simulink model "TIM"  (R2017b)
settings: Solver=ode45  StartTime=0.0  StopTime=inf  RelTol=1e-3
undefined symbols (not defined in the file): sigbuilder_block
(part 1 of 2)
settings Model: Creator=matlab01  LastModifiedBy=matlab01

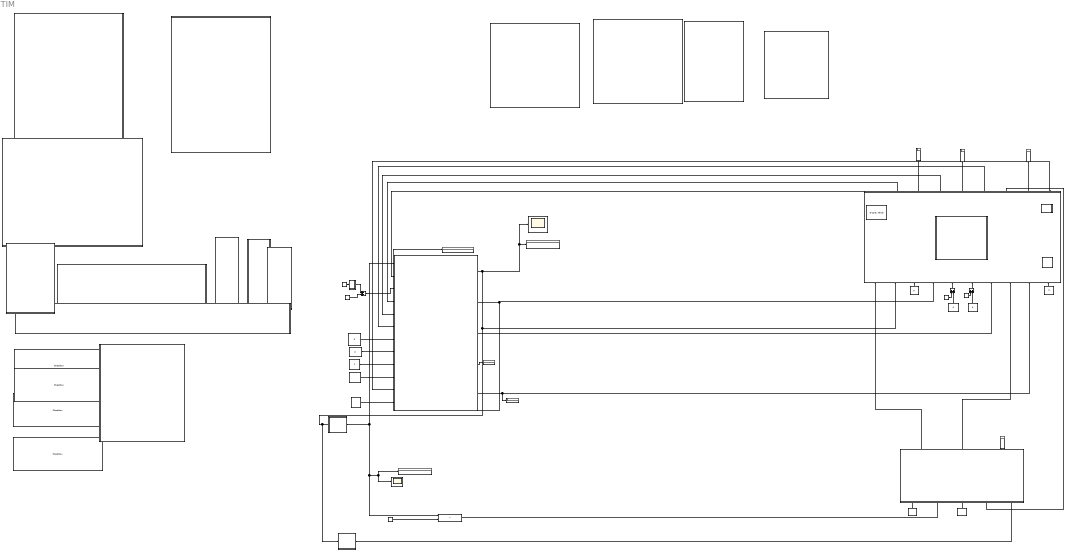
== system TIM ==
  note: Subsystem
  note: Subsystem
  Add : Sum
  Add1 : Sum
  Add2 : Sum
  Bale Pass Sr : Constant  Value=0
  Bale Size Sr : Constant  Value=0
  Baler : Subsystem
  Baler Stopped : Subsystem  DialogController=hmiCreateDDGDialog  IsWebBlock=on  mask(MWDashboardBlock){webBlockId=380f0481-0464-4552-ac21-b39f29efcae4, webBlockType=lamp, ShowInLibBrowser=on, ShowInitialText=on, HMISrcModelName=TIM}
      mask prompts: webBlockType "WebBlock Type"; HMISrcModelName "Source Model"
      mask help: SimulinkHMI:dialogs:LampDialogDesc
      mask Help: helpview([docroot '/mapfiles/simulink.map'], 'hmi_lamp')
      mask Display:
      | if strcmp(get_param(bdroot(gcb),'BlockDiagramType'), 'library')
      |     image([(matlabroot) '/toolbox/simulink/hmi/icons/Lamp.png']);
      | end
  BalerCFG : DisplayBlock  WebBlockId=422  ModelName=TIM  LabelPosition=Hide  ShowInitialText=on  ShowFormattedStrings=off  Format=long  Alignment=Center
  CFG : Display
  Check Box : Checkbox  WebBlockId=680  ModelName=TIM  LabelPosition=Hide  ShowInitialText=off  Checked=on  Label=RearSr_1_Fail
  Check Box1 : Checkbox  WebBlockId=681  ModelName=TIM  LabelPosition=Hide  ShowInitialText=off  Checked=on  Label=RearSr_2_Fail
  Check Box2 : Checkbox  WebBlockId=682  ModelName=TIM  LabelPosition=Hide  ShowInitialText=off  Checked=off  Label=SpeedSr_Fail
  Check Box3 : Checkbox  WebBlockId=683  ModelName=TIM  LabelPosition=Hide  ShowInitialText=off  Checked=off  Label=FrontObstSr_Fail
  Constant : Constant  Value=2
  Constant1 : Constant  Value=2
  Display{,1..2,4..6} (6 alike) : Display
  Display3 : DisplayBlock  WebBlockId=427  ModelName=TIM  LabelPosition=Hide  ShowInitialText=on  ShowFormattedStrings=off  Format=long  Alignment=Center
  Display7 : DisplayBlock  WebBlockId=429  ModelName=TIM  LabelPosition=Hide  ShowInitialText=on  ShowFormattedStrings=off  Format=long  Alignment=Center
  DoorStatus : Display
  Front Obstacle : Constant  Value=0
  FrontObstSr : Subsystem
  FrontObstSrFail : Constant  Value=0
  Gauge : Subsystem  DialogController=hmiCreateDDGDialog  IsWebBlock=on  mask(MWDashboardBlock){webBlockId=a8481909-2d34-4551-932e-729d5791eb58, webBlockType=circulargauge, ShowInLibBrowser=on, ShowInitialText=on, HMISrcModelName=TIM}
      mask prompts: webBlockId "WebBlock Id"; webBlockType "WebBlock Type"; HMISrcModelName "Source Model"
      mask help: SimulinkHMI:dialogs:CircularGaugeDialogDesc
      mask Help: helpview([docroot '/mapfiles/simulink.map'], 'hmi_gauge')
      mask Display:
      | if strcmp(get_param(bdroot(gcb),'BlockDiagramType'), 'library')
      |     image([(matlabroot) '/toolbox/simulink/hmi/icons/CircularGauge.png']);
      | end
  Half Gauge : Subsystem  DialogController=hmiCreateDDGDialog  IsWebBlock=on  mask(MWDashboardBlock){webBlockId=1767aec4-c0de-4876-b9ef-c44c12ba7e5c, webBlockType=semicirculargauge, ShowInLibBrowser=on, ShowInitialText=on, HMISrcModelName=TIM}
      mask prompts: webBlockId "WebBlock Id"; webBlockType "WebBlock Type"; HMISrcModelName "Source Model"
      mask help: SimulinkHMI:dialogs:SemicircularGaugeDialogDesc
      mask Help: helpview([docroot '/mapfiles/simulink.map'], 'hmi_half_gauge')
      mask Display:
      | if strcmp(get_param(bdroot(gcb),'BlockDiagramType'), 'library')
      |     image([(matlabroot) '/toolbox/simulink/hmi/icons/SemicircularGauge.png']);
      | end
  Knob : Subsystem  DialogController=hmiCreateDDGDialog  IsWebBlock=on  mask(MWDashboardBlock){webBlockId=44b2cfbf-7851-438f-9afd-65227a1c2716, webBlockType=continuousknob, ShowInLibBrowser=on, ShowInitialText=on, HMISrcModelName=TIM}
      mask prompts: webBlockId "WebBlock Id"; webBlockType "WebBlock Type"; HMISrcModelName "Source Model"
      mask help: SimulinkHMI:dialogs:ContinuousKnobDialogDesc
      mask Help: helpview([docroot '/mapfiles/simulink.map'], 'hmi_knob')
      mask Display:
      | if strcmp(get_param(bdroot(gcb),'BlockDiagramType'), 'library')
      |     image([(matlabroot) '/toolbox/simulink/hmi/icons/ContinuousKnob.png']);
      | end
  Knob1 : Subsystem  DialogController=hmiCreateDDGDialog  IsWebBlock=on  mask(MWDashboardBlock){webBlockId=555d5953-f540-48b0-b281-3241b1506ee0, webBlockType=continuousknob, ShowInLibBrowser=on, ShowInitialText=on, HMISrcModelName=TIM}
      mask prompts: webBlockId "WebBlock Id"; webBlockType "WebBlock Type"; HMISrcModelName "Source Model"
      mask help: SimulinkHMI:dialogs:ContinuousKnobDialogDesc
      mask Help: helpview([docroot '/mapfiles/simulink.map'], 'hmi_knob')
      mask Display:
      | if strcmp(get_param(bdroot(gcb),'BlockDiagramType'), 'library')
      |     image([(matlabroot) '/toolbox/simulink/hmi/icons/ContinuousKnob.png']);
      | end
  Lamp : Subsystem  DialogController=hmiCreateDDGDialog  IsWebBlock=on  mask(MWDashboardBlock){webBlockId=33d9c165-8687-4e0a-bfea-f4d86ec876ec, webBlockType=lamp, ShowInLibBrowser=on, ShowInitialText=on, HMISrcModelName=TIM}
      mask prompts: webBlockType "WebBlock Type"; HMISrcModelName "Source Model"
      mask help: SimulinkHMI:dialogs:LampDialogDesc
      mask Help: helpview([docroot '/mapfiles/simulink.map'], 'hmi_lamp')
      mask Display:
      | if strcmp(get_param(bdroot(gcb),'BlockDiagramType'), 'library')
      |     image([(matlabroot) '/toolbox/simulink/hmi/icons/Lamp.png']);
      | end
  Lamp1 : Subsystem  DialogController=hmiCreateDDGDialog  IsWebBlock=on  mask(MWDashboardBlock){webBlockId=c492ce9b-3337-4b76-9797-8f79f533d9ec, webBlockType=lamp, ShowInLibBrowser=on, ShowInitialText=on, HMISrcModelName=TIM}
      mask prompts: webBlockType "WebBlock Type"; HMISrcModelName "Source Model"
      mask help: SimulinkHMI:dialogs:LampDialogDesc
      mask Help: helpview([docroot '/mapfiles/simulink.map'], 'hmi_lamp')
      mask Display:
      | if strcmp(get_param(bdroot(gcb),'BlockDiagramType'), 'library')
      |     image([(matlabroot) '/toolbox/simulink/hmi/icons/Lamp.png']);
      | end
  Product : Product
  RearDoor : Subsystem  DialogController=hmiCreateDDGDialog  IsWebBlock=on  mask(MWDashboardBlock){webBlockId=b538fc73-89be-495c-b7c3-b8c3e3397391, webBlockType=lamp, ShowInLibBrowser=on, ShowInitialText=on, HMISrcModelName=TIM}
      mask prompts: webBlockType "WebBlock Type"; HMISrcModelName "Source Model"
      mask help: SimulinkHMI:dialogs:LampDialogDesc
      mask Help: helpview([docroot '/mapfiles/simulink.map'], 'hmi_lamp')
      mask Display:
      | if strcmp(get_param(bdroot(gcb),'BlockDiagramType'), 'library')
      |     image([(matlabroot) '/toolbox/simulink/hmi/icons/Lamp.png']);
      | end
  RearObstSr : Subsystem  DialogController=hmiCreateDDGDialog  IsWebBlock=on  mask(MWDashboardBlock){webBlockId=2f04e0dc-cfdf-4b89-b502-650f31ce5fe2, webBlockType=rockerswitch, ShowInLibBrowser=on, ShowInitialText=on, HMISrcModelName=TIM}
      mask prompts: webBlockId "WebBlock Id"; webBlockType "WebBlock Type"; HMISrcModelName "Source Model"
      mask help: SimulinkHMI:dialogs:SwitchDialogDesc
      mask Help: helpview([docroot '/mapfiles/simulink.map'], 'hmi_rocker_switch')
      mask Display:
      | if strcmp(get_param(bdroot(gcb),'BlockDiagramType'), 'library')
      |     image([(matlabroot) '/toolbox/simulink/hmi/icons/RockerSwitch.png']);
      | end
  RearObstSr1 : Subsystem  DialogController=hmiCreateDDGDialog  IsWebBlock=on  mask(MWDashboardBlock){webBlockId=c64d6447-8e55-46e9-b568-5078a23053e9, webBlockType=rockerswitch, ShowInLibBrowser=on, ShowInitialText=on, HMISrcModelName=TIM}
      mask prompts: webBlockId "WebBlock Id"; webBlockType "WebBlock Type"; HMISrcModelName "Source Model"
      mask help: SimulinkHMI:dialogs:SwitchDialogDesc
      mask Help: helpview([docroot '/mapfiles/simulink.map'], 'hmi_rocker_switch')
      mask Display:
      | if strcmp(get_param(bdroot(gcb),'BlockDiagramType'), 'library')
      |     image([(matlabroot) '/toolbox/simulink/hmi/icons/RockerSwitch.png']);
      | end
  RearObstSr2 : Subsystem  DialogController=hmiCreateDDGDialog  IsWebBlock=on  mask(MWDashboardBlock){webBlockId=c4afeddd-f4a6-4f0c-9e01-adb611532535, webBlockType=rockerswitch, ShowInLibBrowser=on, ShowInitialText=on, HMISrcModelName=TIM}
      mask prompts: webBlockId "WebBlock Id"; webBlockType "WebBlock Type"; HMISrcModelName "Source Model"
      mask help: SimulinkHMI:dialogs:SwitchDialogDesc
      mask Help: helpview([docroot '/mapfiles/simulink.map'], 'hmi_rocker_switch')
      mask Display:
      | if strcmp(get_param(bdroot(gcb),'BlockDiagramType'), 'library')
      |     image([(matlabroot) '/toolbox/simulink/hmi/icons/RockerSwitch.png']);
      | end
  RearSr1 : Constant  Value=0
  RearSr2 : Constant  Value=0
  Rotary Switch : Subsystem  DialogController=hmiCreateDDGDialog  IsWebBlock=on  mask(MWDashboardBlock){webBlockId=4718e849-02b3-481c-8935-c4c34f11cecd, webBlockType=discreteknob, ShowInLibBrowser=on, ShowInitialText=on, HMISrcModelName=TIM}
      mask prompts: webBlockId "WebBlock Id"; webBlockType "WebBlock Type"; HMISrcModelName "Source Model"
      mask help: SimulinkHMI:dialogs:DiscreteKnobDialogDesc
      mask Help: helpview([docroot '/mapfiles/simulink.map'], 'hmi_rotary_switch')
      mask Display:
      | model = bdroot(gcb);
      | if strcmp(get_param(model,'BlockDiagramType'), 'library')
      |     image([(matlabroot) '/toolbox/simulink/hmi/icons/DiscreteKnob.png']);
      | end
  Rotary Switch1 : Subsystem  DialogController=hmiCreateDDGDialog  IsWebBlock=on  mask(MWDashboardBlock){webBlockId=f404cd82-44b9-4011-b588-6289506ab41c, webBlockType=discreteknob, ShowInLibBrowser=on, ShowInitialText=on, HMISrcModelName=TIM}
      mask prompts: webBlockId "WebBlock Id"; webBlockType "WebBlock Type"; HMISrcModelName "Source Model"
      mask help: SimulinkHMI:dialogs:DiscreteKnobDialogDesc
      mask Help: helpview([docroot '/mapfiles/simulink.map'], 'hmi_rotary_switch')
      mask Display:
      | model = bdroot(gcb);
      | if strcmp(get_param(model,'BlockDiagramType'), 'library')
      |     image([(matlabroot) '/toolbox/simulink/hmi/icons/DiscreteKnob.png']);
      | end
  Rotary Switch3 : Subsystem  DialogController=hmiCreateDDGDialog  IsWebBlock=on  mask(MWDashboardBlock){webBlockId=10fa69e3-8ad0-4a7e-b427-115ef8b6ee24, webBlockType=discreteknob, ShowInLibBrowser=on, ShowInitialText=on, HMISrcModelName=TIM}
      mask prompts: webBlockId "WebBlock Id"; webBlockType "WebBlock Type"; HMISrcModelName "Source Model"
      mask help: SimulinkHMI:dialogs:DiscreteKnobDialogDesc
      mask Help: helpview([docroot '/mapfiles/simulink.map'], 'hmi_rotary_switch')
      mask Display:
      | model = bdroot(gcb);
      | if strcmp(get_param(model,'BlockDiagramType'), 'library')
      |     image([(matlabroot) '/toolbox/simulink/hmi/icons/DiscreteKnob.png']);
      | end
  Scope : Scope
  Scope1 : Scope
  SettedSpeed : Display
  Slider : Subsystem  DialogController=hmiCreateDDGDialog  IsWebBlock=on  mask(MWDashboardBlock){webBlockId=15a6815c-0950-4bd8-89d9-de0febee8296, webBlockType=slider, ShowInLibBrowser=on, ShowInitialText=on, HMISrcModelName=TIM}
      mask prompts: webBlockId "WebBlock Id"; webBlockType "WebBlock Type"; HMISrcModelName "Source Model"
      mask help: SimulinkHMI:dialogs:SliderDialogDesc
      mask Help: helpview([docroot '/mapfiles/simulink.map'], 'hmi_slider')
      mask Display:
      | if strcmp(get_param(bdroot(gcb),'BlockDiagramType'), 'library')
      |     image([(matlabroot) '/toolbox/simulink/hmi/icons/Slider.png']);
      | end
  SpSr1Fail : Constant
  "SpeedSr1 " : Subsystem
  SpeedSr2,3 : Subsystem
  SpeedUserInput : Constant  Value=1.6036611567786
  SteeringUserInput : Constant  Value=-8.201570129395
  StopUserCMD : Constant  Value=0
  Swath  Area : Subsystem  DialogController=hmiCreateDDGDialog  IsWebBlock=on  mask(MathWorksWebBlock){webBlockId=664e3edd-25bd-4079-b9dd-da0d72c7846e, webBlockType=continuousknob, ShowInLibBrowser=on, ShowInitialText=on, HMISrcModelName=TIM}
      mask prompts: webBlockId "WebBlock Id"; webBlockType "WebBlock Type"; HMISrcModelName "Source Model"
      mask Help: helpview([docroot '/mapfiles/simulink.map'], 'hmi_knob')
      mask Display:
      | if strcmp(get_param(bdroot(gcb),'BlockDiagramType'), 'library')
      |     image([(matlabroot) '/toolbox/simulink/hmi/icons/ContinuousKnob.png']);
      | end
  Swath Area Value : Constant  Value=4.4148442586263
  SwathLocationSr : Constant  Value=-1.61220043573
  SwathScanner : Subsystem
  SysMode : Constant  Value=3
  Toggle Switch : Subsystem  DialogController=hmiCreateDDGDialog  IsWebBlock=on  mask(MWDashboardBlock){webBlockId=ef49c1b7-d3ac-49f4-96d4-aa01c0f2bdb4, webBlockType=toggleswitch, ShowInLibBrowser=on, ShowInitialText=on, HMISrcModelName=TIM}
      mask prompts: webBlockId "WebBlock Id"; webBlockType "WebBlock Type"; HMISrcModelName "Source Model"
      mask help: SimulinkHMI:dialogs:SwitchDialogDesc
      mask Help: helpview([docroot '/mapfiles/simulink.map'], 'hmi_toggle_switch')
      mask Display:
      | if strcmp(get_param(bdroot(gcb),'BlockDiagramType'), 'library')
      |     image([(matlabroot) '/toolbox/simulink/hmi/icons/ToggleSwitch.png']);
      | end
  Tractor : Subsystem
  ValveUserCMD : Constant
  frontObstSr : Subsystem  DialogController=hmiCreateDDGDialog  IsWebBlock=on  mask(MWDashboardBlock){webBlockId=dd25998f-ff44-4c86-97f2-224d2c2cc3c6, webBlockType=rockerswitch, ShowInLibBrowser=on, ShowInitialText=on, HMISrcModelName=TIM}
      mask prompts: webBlockId "WebBlock Id"; webBlockType "WebBlock Type"; HMISrcModelName "Source Model"
      mask help: SimulinkHMI:dialogs:SwitchDialogDesc
      mask Help: helpview([docroot '/mapfiles/simulink.map'], 'hmi_rocker_switch')
      mask Display:
      | if strcmp(get_param(bdroot(gcb),'BlockDiagramType'), 'library')
      |     image([(matlabroot) '/toolbox/simulink/hmi/icons/RockerSwitch.png']);
      | end
  wires:
  Tractor/1(Speed) -> SpeedSr2,3/1(In1), "SpeedSr1 "/1(In1), Baler/2("settedSpeed "), Scope/1, SettedSpeed/1
  Baler/1(SetSpeedReq) -> Tractor/2(SpeedRequest)
  SwathScanner/1(FlowRate) -> Baler/1(SwathVFlowRate)
  Swath Area Value/1 -> SwathScanner/1(In1)
  Bale Size Sr/1 -> Baler/3(BaleSizeSr)
  Tractor/2(StopCmd) -> Baler/4(StopComand), Display5/1
  Baler/3(StopSign) -> Display4/1
  FrontObstSr/1(Out1) -> Add/1
  Front Obstacle/1 -> FrontObstSr/1(In1)
  Baler/2("StopReq ") -> Tractor/4(StopReq)
  "SpeedSr1 "/1(Out1) -> Tractor/1(currentSpeed), Scope1/1, Display/1, Product/1
  Baler/4(DoorValveReq) -> Tractor/5(ValveReq)
  Bale Pass Sr/1 -> Baler/10(BaleOutSr)
  Tractor/3(Open/CloseCmd) -> Baler/7(RearDoorCmd)
  Baler/5(DoorSign) -> DoorStatus/1
  SwathLocationSr/1 -> SwathScanner/3(SwathLocationSr)
  SwathScanner/2(SwathLocation) -> Baler/8(SwathLocation)
  Tractor/4(SettedAng) -> Display1/1
  Baler/6(SetAngReq) -> Tractor/6(SetAngReq)
  SysMode/1 -> Tractor/7(SysMode)
  Baler/7(RcfgCMD) -> SwathScanner/4(ReCfgCMD)
  Tractor/5("SysModeCmd ") -> Baler/9(ModeCngCMD), Display6/1
  SwathScanner/3(CfgStatus) -> Display2/1
  SpeedSr2,3/1(Out1) -> SwathScanner/5(SpeedSr2,3)
  SpSr1Fail/1 -> Product/2
  Product/1 -> SwathScanner/2(SpeedSr1)
  Add/1 -> Tractor/3(FrontObstSr)
  FrontObstSrFail/1 -> Add/2
  StopUserCMD/1 -> Tractor/8(StopUserInput)
  ValveUserCMD/1 -> Tractor/9(ValveUserInput)
  SpeedUserInput/1 -> Tractor/10(SpeedUserBedal)
  Baler/8(BalerCfg) -> CFG/1
  Add1/1 -> Baler/5(RearObsSr1)
  RearSr1/1 -> Add1/2
  Constant/1 -> Add1/1
  Add2/1 -> Baler/6(RearObstSr2)
  RearSr2/1 -> Add2/2
  Constant1/1 -> Add2/1
  Baler/9(SysReconfigReq) -> Tractor/11("SysReconfigReq ")
  SteeringUserInput/1 -> Tractor/12(SteeringUserInput)

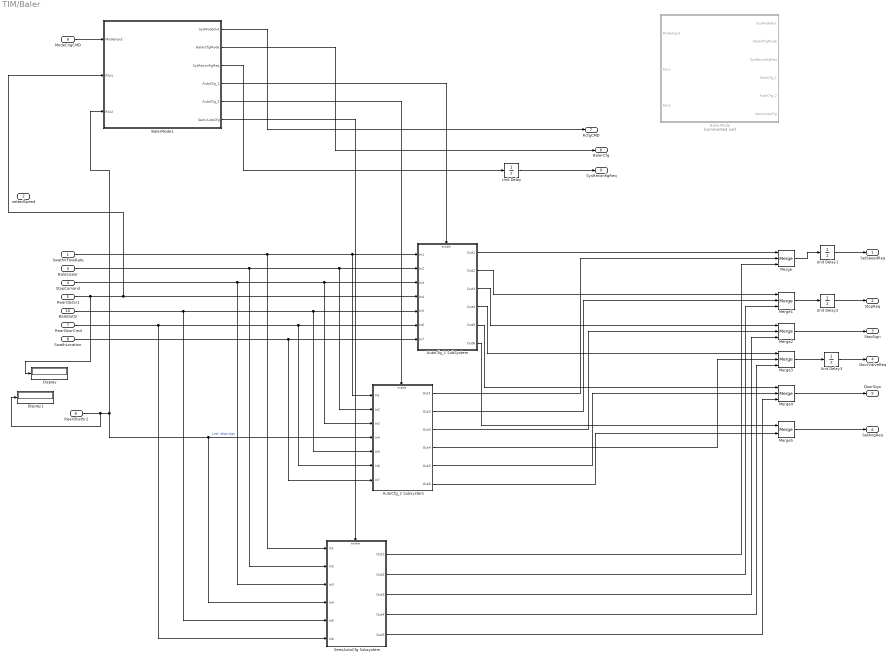
== system TIM/Baler ==
  SwathVFlowRate : Inport
  "settedSpeed " : Inport  Port=2
  BaleSizeSr : Inport  Port=3
  StopComand : Inport  Port=4
  RearObsSr1 : Inport  Port=5
  RearObstSr2 : Inport  Port=6
  RearDoorCmd : Inport  Port=7
  SwathLocation : Inport  Port=8
  ModeCngCMD : Inport  Port=9
  BaleOutSr : Inport  Port=10
  AutoCfg_1 SubSystem : Subsystem
  AutoCfg_2 Subsystem : Subsystem
  BalerMode : Stateflow chart  Commented=on  TreatAsAtomicUnit=on
  BalerMode1 : Stateflow chart  TreatAsAtomicUnit=on
  Display : Display
  Display1 : Display
  Merge{,1..4} (5 alike) : Merge  Inputs=3
  Merge5 : Merge
  SemiAutoCfg Subsystem : Subsystem
  Unit Delay{,1..3} (4 alike) : UnitDelay  SampleTime=-1
  SetSpeedReq : Outport
  "StopReq " : Outport  Port=2
  StopSign : Outport  Port=3
  DoorValveReq : Outport  Port=4
  DoorSign : Outport  Port=5
  SetAngReq : Outport  Port=6
  RcfgCMD : Outport  Port=7
  BalerCfg : Outport  Port=8
  SysReconfigReq : Outport  Port=9
  wires:
  ModeCngCMD/1 -> BalerMode1/1(ModeInput)
  SwathVFlowRate/1 -> SemiAutoCfg Subsystem/1(In1), AutoCfg_2 Subsystem/1(In1), AutoCfg_1 SubSystem/1(In1)
  BaleSizeSr/1 -> SemiAutoCfg Subsystem/2(In2), AutoCfg_2 Subsystem/2(In2), AutoCfg_1 SubSystem/2(In2)
  StopComand/1 -> SemiAutoCfg Subsystem/3(In3), AutoCfg_2 Subsystem/3(In3), AutoCfg_1 SubSystem/3(In3)  "just  stop sign"
  RearObsSr1/1 -> Display/1, BalerMode1/2(RSr1), AutoCfg_1 SubSystem/4(In4)
  BaleOutSr/1 -> SemiAutoCfg Subsystem/5(In5), AutoCfg_2 Subsystem/5(In5), AutoCfg_1 SubSystem/5(In5)
  RearDoorCmd/1 -> SemiAutoCfg Subsystem/6(In6), AutoCfg_2 Subsystem/6(In6), AutoCfg_1 SubSystem/6(In6)
  SwathLocation/1 -> AutoCfg_1 SubSystem/7(In7), AutoCfg_2 Subsystem/7(In7)
  AutoCfg_1 SubSystem/3(Out3) -> Merge2/1
  AutoCfg_1 SubSystem/6(Out6) -> Merge5/1
  RearObstSr2/1 -> Display1/1, BalerMode1/3(RSr2), SemiAutoCfg Subsystem/4(In4), AutoCfg_2 Subsystem/4(In4)
  BalerMode1/1(SysModeOut) -> RcfgCMD/1
  BalerMode1/3(SysReconfigReq) -> Unit Delay/1
  Unit Delay/1 -> SysReconfigReq/1
  BalerMode1/4(AutoCfg_1) -> AutoCfg_1 SubSystem/Enable
  BalerMode1/5(AutoCfg_2) -> AutoCfg_2 Subsystem/Enable
  Merge/1 -> Unit Delay1/1
  Merge1/1 -> Unit Delay2/1
  Merge2/1 -> StopSign/1
  Merge3/1 -> Unit Delay3/1
  Merge4/1 -> DoorSign/1
  Merge5/1 -> SetAngReq/1
  AutoCfg_2 Subsystem/3(Out3) -> Merge2/2
  AutoCfg_1 SubSystem/5(Out5) -> Merge4/1
  AutoCfg_2 Subsystem/5(Out5) -> Merge4/2
  AutoCfg_2 Subsystem/6(Out6) -> Merge5/2
  AutoCfg_1 SubSystem/1(Out1) -> Merge/1
  AutoCfg_1 SubSystem/2(Out2) -> Merge1/1
  AutoCfg_1 SubSystem/4(Out4) -> Merge3/1
  AutoCfg_2 Subsystem/1(Out1) -> Merge/2
  AutoCfg_2 Subsystem/2(Out2) -> Merge1/2
  AutoCfg_2 Subsystem/4(Out4) -> Merge3/2
  Unit Delay1/1 -> SetSpeedReq/1
  Unit Delay2/1 -> "StopReq "/1
  Unit Delay3/1 -> DoorValveReq/1
  SemiAutoCfg Subsystem/1(Out1) -> Merge/3
  SemiAutoCfg Subsystem/2(Out2) -> Merge1/3
  SemiAutoCfg Subsystem/3(Out3) -> Merge2/3
  SemiAutoCfg Subsystem/4(Out4) -> Merge3/3
  SemiAutoCfg Subsystem/5(Out5) -> Merge4/3
  BalerMode1/6(SemiAutoCfg) -> SemiAutoCfg Subsystem/Enable
  BalerMode1/2(BalerCfgMode) -> BalerCfg/1

== system TIM/Baler Stopped ==

== system TIM/FrontObstSr ==
  In1 : Inport
  Data Type Conversion : DataTypeConversion  OutDataTypeStr=boolean
  Out1 : Outport
  wires:
  In1/1 -> Data Type Conversion/1
  Data Type Conversion/1 -> Out1/1

== system TIM/Gauge ==

== system TIM/Half Gauge ==

== system TIM/Knob ==

== system TIM/Knob1 ==

== system TIM/Lamp ==

== system TIM/Lamp1 ==

== system TIM/RearDoor ==

== system TIM/RearObstSr ==

== system TIM/RearObstSr1 ==

== system TIM/RearObstSr2 ==

== system TIM/Rotary Switch ==

== system TIM/Rotary Switch1 ==

== system TIM/Rotary Switch3 ==

== system TIM/Slider ==

== system TIM/SpeedSr1  ==
  In1 : Inport
  Signal Builder1 : Subsystem  Tag=STV Subsys  LoadFcn=sigbuilder_block('load');  StartFcn=sigbuilder_block('start');  StopFcn=sigbuilder_block('stop');  ClipboardFcn=sigbuilder_block('clipboard');  mask(Sigbuilder block){tuvar=[0:10]}
      mask help: Simulink:masks:SigbuilderBlock_MD
      mask init:
      | if ~strcmp(get_param(bdroot(gcbh),'SimulationStatus'),'stopped') tuvar = sigbuilder_block('maskInit'); end
      settings: CopyFcn=sigbuilder_block('copy');  DeleteFcn=sigbuilder_block('delete');  ModelCloseFcn=sigbuilder_block('modelClose');  PreSaveFcn=sigbuilder_block('preSave');  PauseFcn=sigbuilder_block('pause');  ContinueFcn=sigbuilder_block('continue');  NameChangeFcn=sigbuilder_block('namechange');  OpenFcn=sigbuilder_block('open',[438.75 215.25 544.5 355.5 ]);  CloseFcn=sigbuilder_block('close');
      mask Display: plot(0, 0, 100, 100,[2, 2, 32, 32, 2], [68, 8, 8, 68, 68],[32, 2], [38, 38], [32, 19, 2],[53, 60, 44], [32, 17, 17, 2],[16, 16, 31, 31]);txt = getActiveGroup(gcbh);text(2, 100, txt,'verticalAlignment', 'top');
  Switch : Switch  Threshold=8
  Unit Delay : UnitDelay  SampleTime=-1
  Out1 : Outport
  wires:
  Signal Builder1/1(Signal 1) -> Switch/3, Switch/2
  In1/1 -> Unit Delay/1
  Switch/1 -> Out1/1
  Unit Delay/1 -> Switch/1

== system TIM/SpeedSr2,3 ==
  In1 : Inport
  Signal Builder1 : Subsystem  Tag=STV Subsys  LoadFcn=sigbuilder_block('load');  StartFcn=sigbuilder_block('start');  StopFcn=sigbuilder_block('stop');  ClipboardFcn=sigbuilder_block('clipboard');  mask(Sigbuilder block){tuvar=[0:10]}
      mask help: Simulink:masks:SigbuilderBlock_MD
      mask init:
      | if ~strcmp(get_param(bdroot(gcbh),'SimulationStatus'),'stopped') tuvar = sigbuilder_block('maskInit'); end
      settings: CopyFcn=sigbuilder_block('copy');  DeleteFcn=sigbuilder_block('delete');  ModelCloseFcn=sigbuilder_block('modelClose');  PreSaveFcn=sigbuilder_block('preSave');  PauseFcn=sigbuilder_block('pause');  ContinueFcn=sigbuilder_block('continue');  NameChangeFcn=sigbuilder_block('namechange');  OpenFcn=sigbuilder_block('open',[438.75 215.25 544.5 355.5 ]);  CloseFcn=sigbuilder_block('close');
      mask Display: plot(0, 0, 100, 100,[2, 2, 32, 32, 2], [68, 8, 8, 68, 68],[32, 2], [38, 38], [32, 19, 2],[53, 60, 44], [32, 17, 17, 2],[16, 16, 31, 31]);txt = getActiveGroup(gcbh);text(2, 100, txt,'verticalAlignment', 'top');
  Switch : Switch  Threshold=8
  Out1 : Outport
  wires:
  In1/1 -> Switch/1
  Switch/1 -> Out1/1
  Signal Builder1/1(Signal 1) -> Switch/2, Switch/3

== system TIM/Swath  Area ==

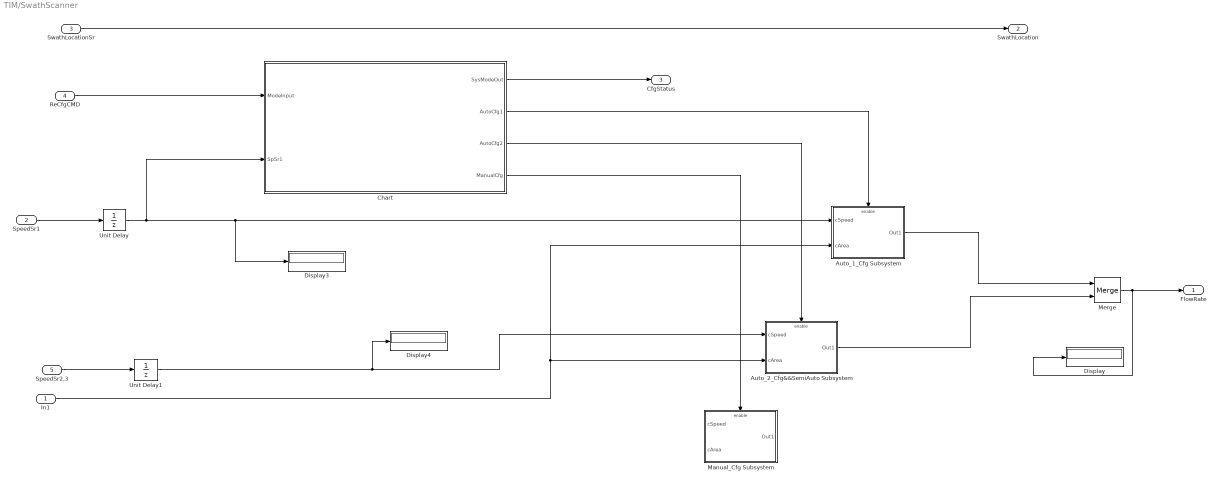
== system TIM/SwathScanner ==
  In1 : Inport
  SpeedSr1 : Inport  Port=2
  SwathLocationSr : Inport  Port=3
  ReCfgCMD : Inport  Port=4
  SpeedSr2,3 : Inport  Port=5
  Auto_1_Cfg Subsystem : Subsystem  TreatAsAtomicUnit=on
  Auto_2_Cfg&&SemiAuto Subsystem : Subsystem  TreatAsAtomicUnit=on
  Chart : Stateflow chart  TreatAsAtomicUnit=on
  Display : Display
  Display3 : Display
  Display4 : Display
  Manual_Cfg Subsystem : Subsystem  TreatAsAtomicUnit=on
  Merge : Merge
  Unit Delay : UnitDelay  SampleTime=-1
  Unit Delay1 : UnitDelay  SampleTime=-1
  FlowRate : Outport
  SwathLocation : Outport  Port=2
  CfgStatus : Outport  Port=3
  wires:
  ReCfgCMD/1 -> Chart/1(ModeInput)
  Chart/1(SysModeOut) -> CfgStatus/1
  Auto_2_Cfg&&SemiAuto Subsystem/1(Out1) -> Merge/2
  SpeedSr2,3/1 -> Unit Delay1/1
  In1/1 -> Auto_1_Cfg Subsystem/2(cArea), Auto_2_Cfg&&SemiAuto Subsystem/2(cArea)
  Auto_1_Cfg Subsystem/1(Out1) -> Merge/1
  Unit Delay/1 -> Chart/2(SpSr1), Display3/1, Auto_1_Cfg Subsystem/1(cSpeed)
  SwathLocationSr/1 -> SwathLocation/1
  Merge/1 -> Display/1, FlowRate/1
  Unit Delay1/1 -> Display4/1, Auto_2_Cfg&&SemiAuto Subsystem/1(cSpeed)
  SpeedSr1/1 -> Unit Delay/1
  Chart/2(AutoCfg1) -> Auto_1_Cfg Subsystem/Enable
  Chart/3(AutoCfg2) -> Auto_2_Cfg&&SemiAuto Subsystem/Enable
  Chart/4(ManualCfg) -> Manual_Cfg Subsystem/Enable

== system TIM/Toggle Switch ==

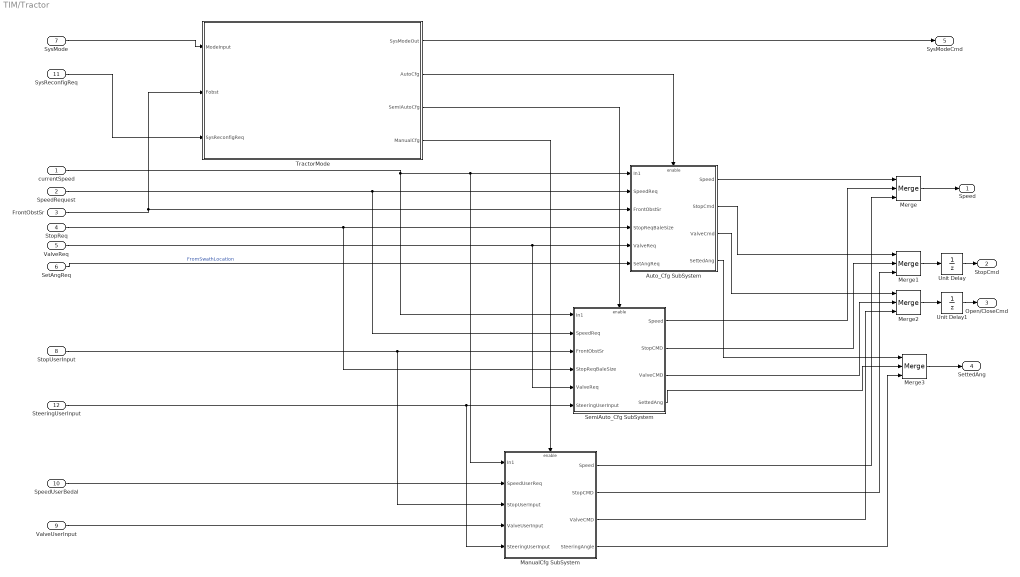
== system TIM/Tractor ==
  currentSpeed : Inport
  SpeedRequest : Inport  Port=2
  FrontObstSr : Inport  Port=3
  StopReq : Inport  Port=4
  ValveReq : Inport  Port=5
  SetAngReq : Inport  Port=6
  SysMode : Inport  Port=7
  StopUserInput : Inport  Port=8
  ValveUserInput : Inport  Port=9
  SpeedUserBedal : Inport  Port=10
  "SysReconfigReq " : Inport  Port=11
  SteeringUserInput : Inport  Port=12
  Auto_Cfg SubSystem : Subsystem
  ManualCfg SubSystem : Subsystem
  Merge{,1..3} (4 alike) : Merge  Inputs=3
  SemiAuto_Cfg SubSystem : Subsystem
  TractorMode : Stateflow chart  TreatAsAtomicUnit=on
  Unit Delay : UnitDelay  SampleTime=-1
  Unit Delay1 : UnitDelay  SampleTime=-1
  Speed : Outport
  StopCmd : Outport  Port=2
  Open/CloseCmd : Outport  Port=3
  SettedAng : Outport  Port=4
  "SysModeCmd " : Outport  Port=5
  wires:
  FrontObstSr/1 -> TractorMode/2(Fobst), Auto_Cfg SubSystem/3(FrontObstSr)
  SetAngReq/1 -> Auto_Cfg SubSystem/6(SetAngReq)  "FromSwathLocation"
  SysMode/1 -> TractorMode/1(ModeInput)
  TractorMode/1(SysModeOut) -> "SysModeCmd "/1
  currentSpeed/1 -> SemiAuto_Cfg SubSystem/1(In1), ManualCfg SubSystem/1(In1), Auto_Cfg SubSystem/1(In1)
  SpeedRequest/1 -> SemiAuto_Cfg SubSystem/2(SpeedReq), Auto_Cfg SubSystem/2(SpeedReq)
  StopReq/1 -> SemiAuto_Cfg SubSystem/4(StopReqBaleSize), Auto_Cfg SubSystem/4(StopReqBaleSize)
  ValveReq/1 -> SemiAuto_Cfg SubSystem/5(ValveReq), Auto_Cfg SubSystem/5(ValveReq)
  StopUserInput/1 -> ManualCfg SubSystem/3(StopUserInput), SemiAuto_Cfg SubSystem/3(FrontObstSr)
  TractorMode/2(AutoCfg) -> Auto_Cfg SubSystem/Enable
  TractorMode/3(SemiAutoCfg) -> SemiAuto_Cfg SubSystem/Enable
  SemiAuto_Cfg SubSystem/1(Speed) -> Merge/2
  SemiAuto_Cfg SubSystem/2(StopCMD) -> Merge1/2
  SemiAuto_Cfg SubSystem/3(ValveCMD) -> Merge2/2
  Auto_Cfg SubSystem/1(Speed) -> Merge/1
  Merge/1 -> Speed/1
  Merge1/1 -> Unit Delay/1
  Merge2/1 -> Unit Delay1/1
  Auto_Cfg SubSystem/2(StopCmd) -> Merge1/1
  Auto_Cfg SubSystem/3(ValveCmd) -> Merge2/1
  TractorMode/4(ManualCfg) -> ManualCfg SubSystem/Enable
  SpeedUserBedal/1 -> ManualCfg SubSystem/2(SpeedUserReq)
  ValveUserInput/1 -> ManualCfg SubSystem/4(ValveUserInput)
  ManualCfg SubSystem/1(Speed) -> Merge/3
  "SysReconfigReq "/1 -> TractorMode/3(SysReconfigReq)
  SteeringUserInput/1 -> ManualCfg SubSystem/5(SteeringUserInput), SemiAuto_Cfg SubSystem/6(SteeringUserInput)
  ManualCfg SubSystem/2(StopCMD) -> Merge1/3
  ManualCfg SubSystem/3(ValveCMD) -> Merge2/3
  Merge3/1 -> SettedAng/1
  Auto_Cfg SubSystem/4(SettedAng) -> Merge3/1
  SemiAuto_Cfg SubSystem/4(SettedAng) -> Merge3/2
  ManualCfg SubSystem/4(SteeringAngle) -> Merge3/3
  Unit Delay/1 -> StopCmd/1
  Unit Delay1/1 -> Open/CloseCmd/1

== system TIM/frontObstSr ==

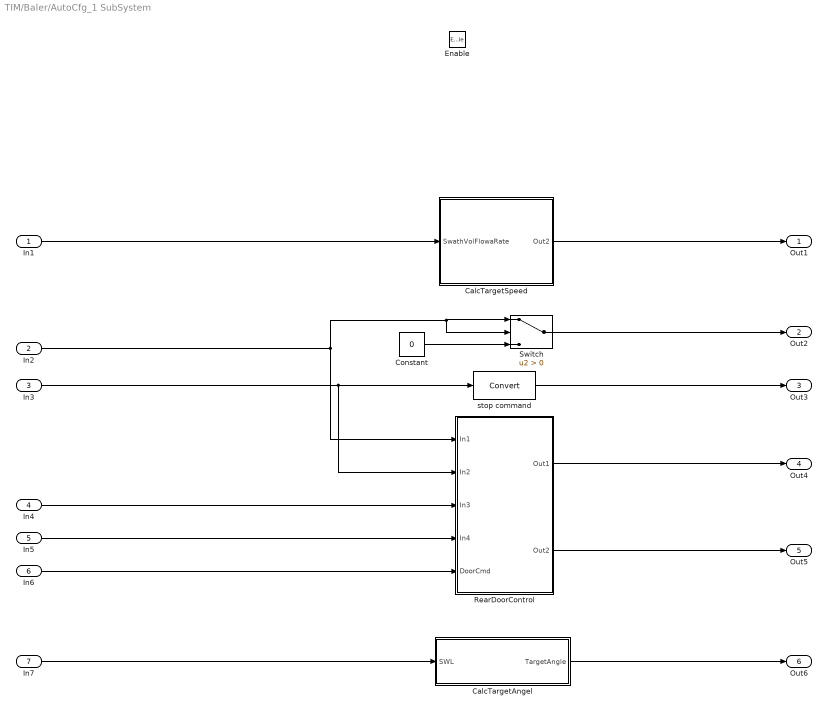
== system TIM/Baler/AutoCfg_1 SubSystem ==
  In1 : Inport
  In2 : Inport  Port=2
  In3 : Inport  Port=3
  In4 : Inport  Port=4
  In5 : Inport  Port=5
  In6 : Inport  Port=6
  In7 : Inport  Port=7
  Enable : EnablePort
  CalcTargetAngel : MATLAB Function  TreatAsAtomicUnit=on
  CalcTargetSpeed : Subsystem
  Constant : Constant  Value=0
  RearDoorControl : Subsystem
  Switch : Switch  Criteria=u2 > Threshold
  stop command : DataTypeConversion
  Out1 : Outport
  Out2 : Outport  Port=2
  Out3 : Outport  Port=3
  Out4 : Outport  Port=4
  Out5 : Outport  Port=5
  Out6 : Outport  Port=6
  wires:
  CalcTargetSpeed/1(Out2) -> Out1/1
  In1/1 -> CalcTargetSpeed/1(SwathVolFlowaRate)
  Switch/1 -> Out2/1
  In6/1 -> RearDoorControl/5(DoorCmd)
  stop command/1 -> Out3/1
  RearDoorControl/1(Out1) -> Out4/1
  In7/1 -> CalcTargetAngel/1(SWL)
  In4/1 -> RearDoorControl/3(In3)
  In5/1 -> RearDoorControl/4(In4)
  In3/1 -> stop command/1, RearDoorControl/2(In2)
  In2/1 -> Switch/2, Switch/1, RearDoorControl/1(In1)
  RearDoorControl/2(Out2) -> Out5/1
  CalcTargetAngel/1(TargetAngle) -> Out6/1
  Constant/1 -> Switch/3

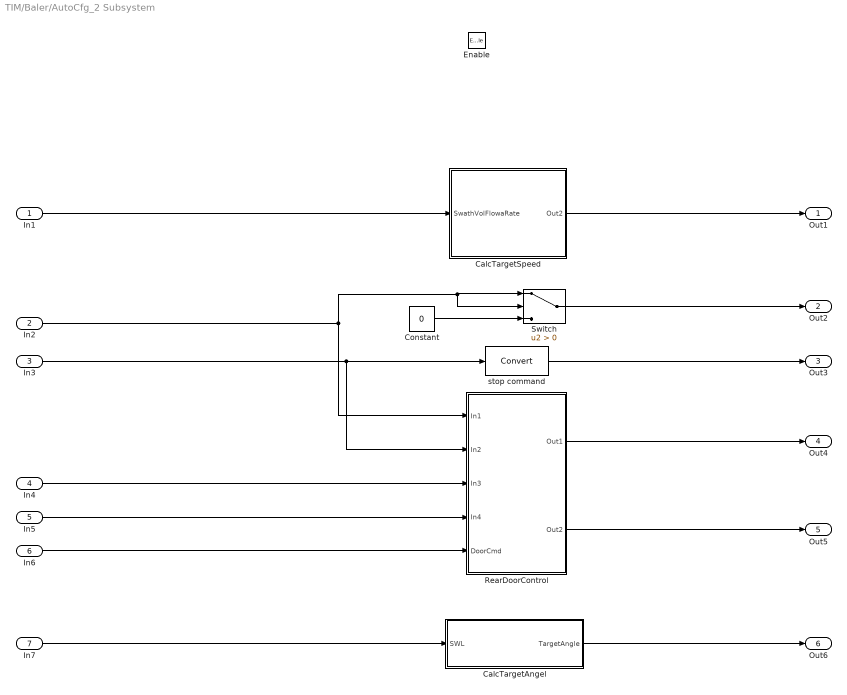
== system TIM/Baler/AutoCfg_2 Subsystem ==
  In1 : Inport
  In2 : Inport  Port=2
  In3 : Inport  Port=3
  In4 : Inport  Port=4
  In5 : Inport  Port=5
  In6 : Inport  Port=6
  In7 : Inport  Port=7
  Enable : EnablePort
  CalcTargetAngel : MATLAB Function  TreatAsAtomicUnit=on
  CalcTargetSpeed : Subsystem
  Constant : Constant  Value=0
  RearDoorControl : Subsystem
  Switch : Switch  Criteria=u2 > Threshold
  stop command : DataTypeConversion
  Out1 : Outport
  Out2 : Outport  Port=2
  Out3 : Outport  Port=3
  Out4 : Outport  Port=4
  Out5 : Outport  Port=5
  Out6 : Outport  Port=6
  wires:
  Constant/1 -> Switch/3
  CalcTargetAngel/1(TargetAngle) -> Out6/1
  RearDoorControl/2(Out2) -> Out5/1
  In2/1 -> RearDoorControl/1(In1), Switch/1, Switch/2
  In3/1 -> RearDoorControl/2(In2), stop command/1
  In5/1 -> RearDoorControl/4(In4)
  In4/1 -> RearDoorControl/3(In3)
  In7/1 -> CalcTargetAngel/1(SWL)
  RearDoorControl/1(Out1) -> Out4/1
  stop command/1 -> Out3/1
  In6/1 -> RearDoorControl/5(DoorCmd)
  Switch/1 -> Out2/1
  In1/1 -> CalcTargetSpeed/1(SwathVolFlowaRate)
  CalcTargetSpeed/1(Out2) -> Out1/1

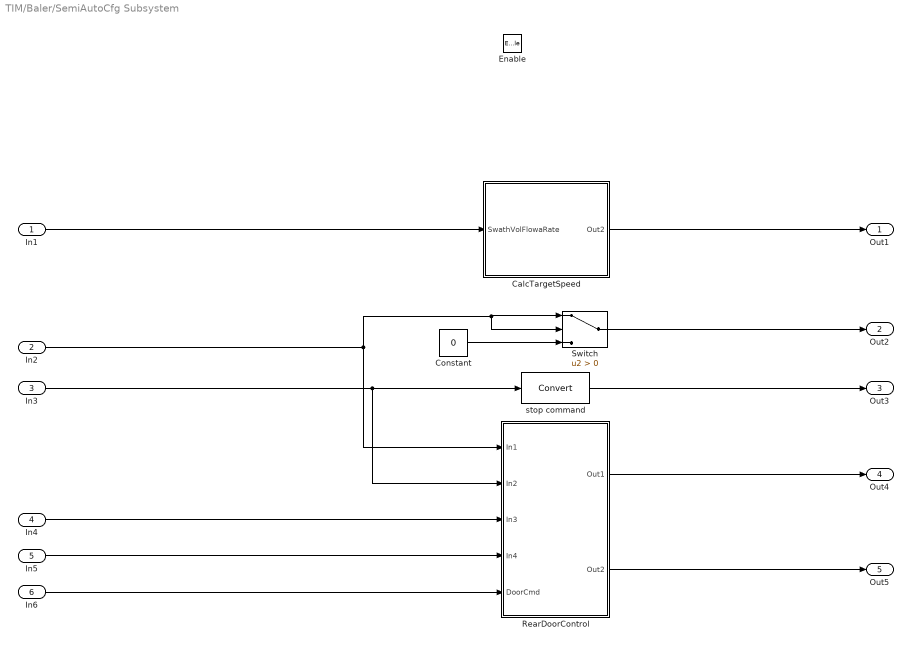
== system TIM/Baler/SemiAutoCfg Subsystem ==
  In1 : Inport
  In2 : Inport  Port=2
  In3 : Inport  Port=3
  In4 : Inport  Port=4
  In5 : Inport  Port=5
  In6 : Inport  Port=6
  Enable : EnablePort
  CalcTargetSpeed : Subsystem
  Constant : Constant  Value=0
  RearDoorControl : Subsystem
  Switch : Switch  Criteria=u2 > Threshold
  stop command : DataTypeConversion
  Out1 : Outport
  Out2 : Outport  Port=2
  Out3 : Outport  Port=3
  Out4 : Outport  Port=4
  Out5 : Outport  Port=5
  wires:
  CalcTargetSpeed/1(Out2) -> Out1/1
  In1/1 -> CalcTargetSpeed/1(SwathVolFlowaRate)
  Switch/1 -> Out2/1
  In6/1 -> RearDoorControl/5(DoorCmd)
  stop command/1 -> Out3/1
  RearDoorControl/1(Out1) -> Out4/1
  In4/1 -> RearDoorControl/3(In3)
  In5/1 -> RearDoorControl/4(In4)
  In3/1 -> stop command/1, RearDoorControl/2(In2)
  In2/1 -> Switch/2, Switch/1, RearDoorControl/1(In1)
  RearDoorControl/2(Out2) -> Out5/1
  Constant/1 -> Switch/3

== system TIM/SpeedSr1 /Signal Builder1 ==
  Demux : Demux  Tag=STV Demux  Outputs=1
  FromWs : FromWorkspace  Tag=STV FromWs  VariableName=tuvar  SampleTime=0
      SigBuilderData=|
      | common.afterFinalStr = 'Extrapolate'
      | common.sampleTime = 0
      | dataSet.timeRange = [0 20]
      | dataSet.name = 'Group 1'
      | sbobj.Groups.Name = 'Group 1'
      | sbobj.Groups.Signals.Name = 'Signal 1'
      | sbobj.Groups.Signals.XData = [0 4 6 8 10 20]
      | sbobj.Groups.Signals.YData = [0 4 5.95 10 10 10]
      | sbobj.Groups.TimeRange = [0 20]
  Signal 1 : Outport  Tag=STV Outport
  wires:
  Demux/1 -> Signal 1/1
  FromWs/1 -> Demux/1

== system TIM/SpeedSr2,3/Signal Builder1 ==
  Demux : Demux  Tag=STV Demux  Outputs=1
  FromWs : FromWorkspace  Tag=STV FromWs  VariableName=tuvar  SampleTime=0
      SigBuilderData=|
      | common.afterFinalStr = 'Extrapolate'
      | common.sampleTime = 0
      | dataSet.timeRange = [0 20]
      | dataSet.name = 'Group 1'
      | sbobj.Groups.Name = 'Group 1'
      | sbobj.Groups.Signals.Name = 'Signal 1'
      | sbobj.Groups.Signals.XData = [0 4 6 8 10 20]
      | sbobj.Groups.Signals.YData = [0 4 5.95 10 10 10]
      | sbobj.Groups.TimeRange = [0 20]
  Signal 1 : Outport  Tag=STV Outport
  wires:
  FromWs/1 -> Demux/1
  Demux/1 -> Signal 1/1

== system TIM/SwathScanner/Auto_1_Cfg Subsystem ==
  cSpeed : Inport
  cArea : Inport  Port=2
  Enable : EnablePort  StatesWhenEnabling=reset
  CalcVolFlowRate 1 : Subsystem
  Out1 : Outport
  wires:
  cSpeed/1 -> CalcVolFlowRate 1/1(CurrentSpeed)
  CalcVolFlowRate 1/1(Out1) -> Out1/1
  cArea/1 -> CalcVolFlowRate 1/2(SwathArea)

== system TIM/SwathScanner/Auto_2_Cfg&&SemiAuto Subsystem ==
  cSpeed : Inport
  cArea : Inport  Port=2
  Enable : EnablePort
  CalcVolFlowRate 1 : Subsystem
  Out1 : Outport
  wires:
  cArea/1 -> CalcVolFlowRate 1/2(SwathArea)
  CalcVolFlowRate 1/1(Out1) -> Out1/1
  cSpeed/1 -> CalcVolFlowRate 1/1(CurrentSpeed)

== system TIM/SwathScanner/Manual_Cfg Subsystem ==
  cSpeed : Inport
  cArea : Inport  Port=2
  Enable : EnablePort
  CalcVolFlowRate 1 : Subsystem
  Out1 : Outport
  wires:
  cSpeed/1 -> CalcVolFlowRate 1/1(CurrentSpeed)
  CalcVolFlowRate 1/1(Out1) -> Out1/1
  cArea/1 -> CalcVolFlowRate 1/2(SwathArea)

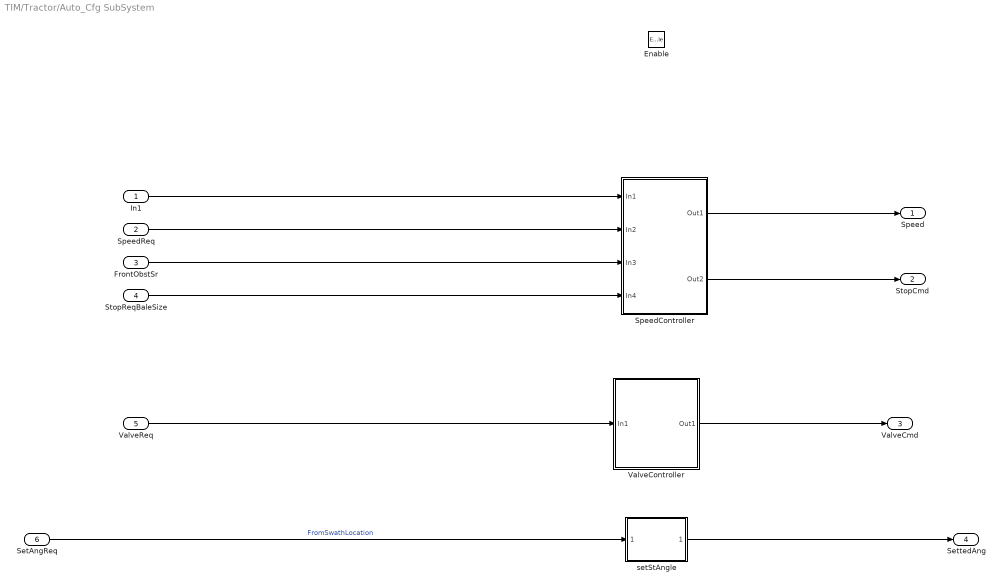
== system TIM/Tractor/Auto_Cfg SubSystem ==
  In1 : Inport
  SpeedReq : Inport  Port=2
  FrontObstSr : Inport  Port=3
  StopReqBaleSize : Inport  Port=4
  ValveReq : Inport  Port=5
  SetAngReq : Inport  Port=6
  Enable : EnablePort
  SpeedController : Subsystem
  ValveController : Subsystem
  setStAngle : MATLAB Function  TreatAsAtomicUnit=on
  Speed : Outport
  StopCmd : Outport  Port=2
  ValveCmd : Outport  Port=3
  SettedAng : Outport  Port=4
  wires:
  FrontObstSr/1 -> SpeedController/3(In3)
  SpeedReq/1 -> SpeedController/2(In2)
  SpeedController/2(Out2) -> StopCmd/1
  ValveController/1(Out1) -> ValveCmd/1
  ValveReq/1 -> ValveController/1(In1)
  SpeedController/1(Out1) -> Speed/1
  StopReqBaleSize/1 -> SpeedController/4(In4)
  In1/1 -> SpeedController/1(In1)
  SetAngReq/1 -> setStAngle/1(TAngle)  "FromSwathLocation"
  setStAngle/1(CAngle) -> SettedAng/1

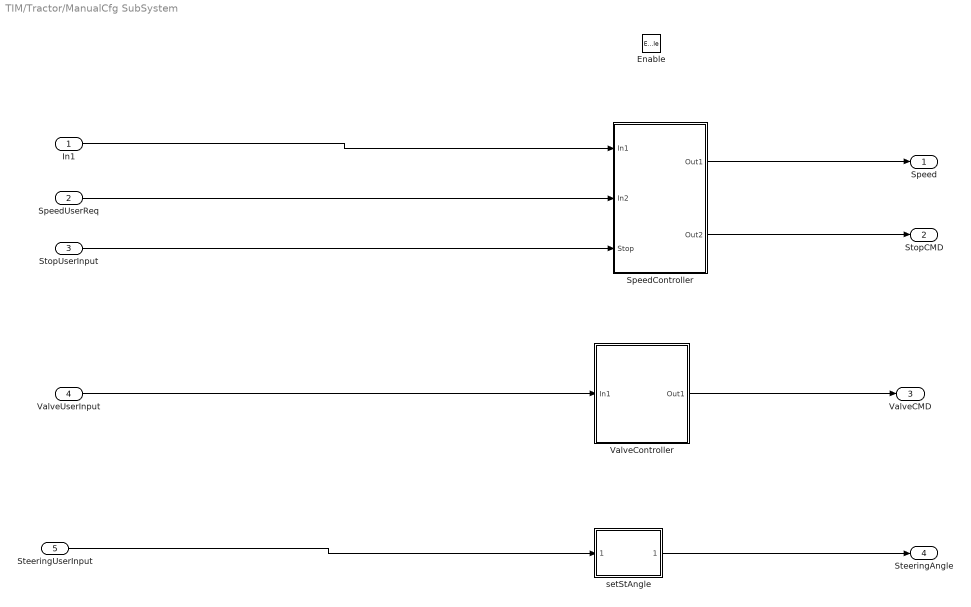
== system TIM/Tractor/ManualCfg SubSystem ==
  In1 : Inport
  SpeedUserReq : Inport  Port=2
  StopUserInput : Inport  Port=3
  ValveUserInput : Inport  Port=4
  SteeringUserInput : Inport  Port=5
  Enable : EnablePort
  SpeedController : Subsystem
  ValveController : Subsystem
  setStAngle : MATLAB Function  TreatAsAtomicUnit=on
  Speed : Outport
  StopCMD : Outport  Port=2
  ValveCMD : Outport  Port=3
  SteeringAngle : Outport  Port=4
  wires:
  StopUserInput/1 -> SpeedController/3(Stop)
  SpeedUserReq/1 -> SpeedController/2(In2)
  SpeedController/2(Out2) -> StopCMD/1
  ValveController/1(Out1) -> ValveCMD/1
  ValveUserInput/1 -> ValveController/1(In1)
  SpeedController/1(Out1) -> Speed/1
  In1/1 -> SpeedController/1(In1)
  SteeringUserInput/1 -> setStAngle/1(TAngle)
  setStAngle/1(CAngle) -> SteeringAngle/1

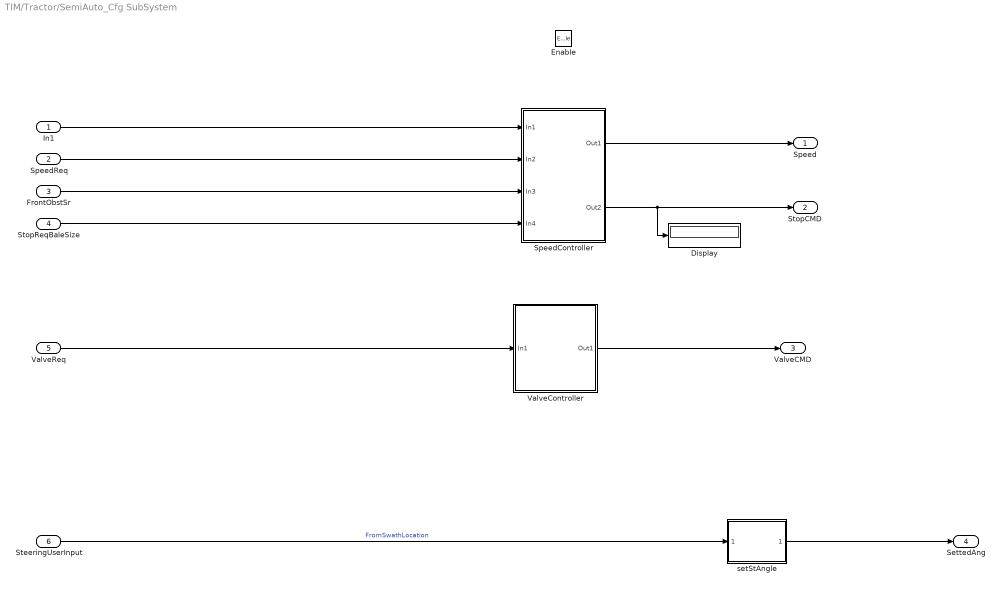
== system TIM/Tractor/SemiAuto_Cfg SubSystem ==
  In1 : Inport
  SpeedReq : Inport  Port=2
  FrontObstSr : Inport  Port=3
  StopReqBaleSize : Inport  Port=4
  ValveReq : Inport  Port=5
  SteeringUserInput : Inport  Port=6
  Enable : EnablePort
  Display : Display
  SpeedController : Subsystem
  ValveController : Subsystem
  setStAngle : MATLAB Function  TreatAsAtomicUnit=on
  Speed : Outport
  StopCMD : Outport  Port=2
  ValveCMD : Outport  Port=3
  SettedAng : Outport  Port=4
  wires:
  In1/1 -> SpeedController/1(In1)
  StopReqBaleSize/1 -> SpeedController/4(In4)
  SpeedController/1(Out1) -> Speed/1
  ValveReq/1 -> ValveController/1(In1)
  ValveController/1(Out1) -> ValveCMD/1
  SpeedController/2(Out2) -> Display/1, StopCMD/1
  SpeedReq/1 -> SpeedController/2(In2)
  FrontObstSr/1 -> SpeedController/3(In3)
  SteeringUserInput/1 -> setStAngle/1(TAngle)  "FromSwathLocation"
  setStAngle/1(CAngle) -> SettedAng/1

== system TIM/Baler/AutoCfg_1 SubSystem/CalcTargetSpeed ==
  SwathVolFlowaRate : Inport
  MATLAB Function : MATLAB Function  TreatAsAtomicUnit=on
  Out2 : Outport
  wires:
  SwathVolFlowaRate/1 -> MATLAB Function/1(u)
  MATLAB Function/1(TargetSpeed) -> Out2/1

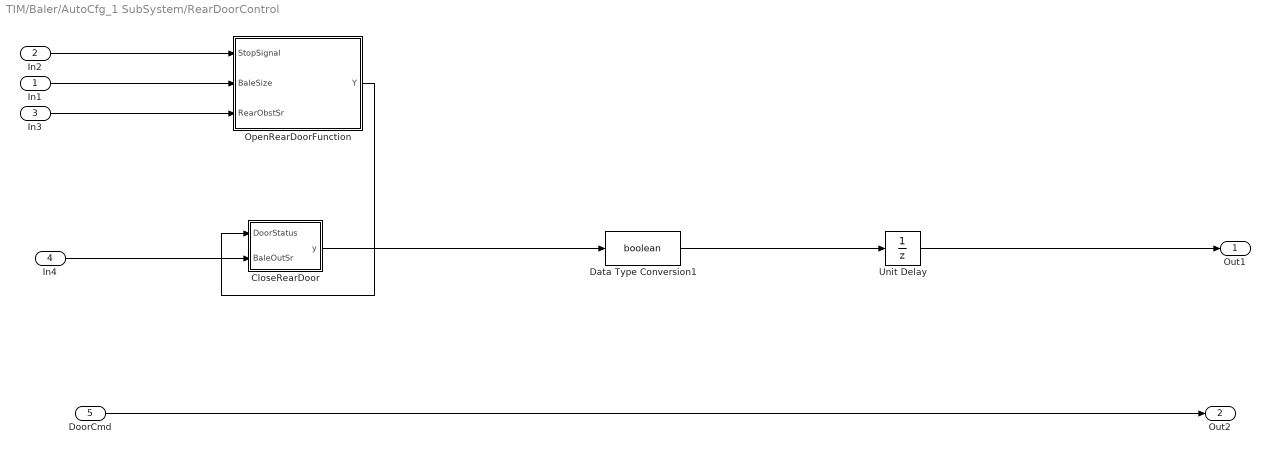
== system TIM/Baler/AutoCfg_1 SubSystem/RearDoorControl ==
  In1 : Inport
  In2 : Inport  Port=2
  In3 : Inport  Port=3
  In4 : Inport  Port=4
  DoorCmd : Inport  Port=5
  CloseRearDoor : MATLAB Function  TreatAsAtomicUnit=on
  Data Type Conversion1 : DataTypeConversion  OutDataTypeStr=boolean
  OpenRearDoorFunction : MATLAB Function  TreatAsAtomicUnit=on
  Unit Delay : UnitDelay  SampleTime=-1
  Out1 : Outport
  Out2 : Outport  Port=2
  wires:
  CloseRearDoor/1(y) -> Data Type Conversion1/1
  In3/1 -> OpenRearDoorFunction/3(RearObstSr)
  OpenRearDoorFunction/1(Y) -> CloseRearDoor/1(DoorStatus)
  Data Type Conversion1/1 -> Unit Delay/1
  In1/1 -> OpenRearDoorFunction/2(BaleSize)
  In2/1 -> OpenRearDoorFunction/1(StopSignal)
  In4/1 -> CloseRearDoor/2(BaleOutSr)
  DoorCmd/1 -> Out2/1
  Unit Delay/1 -> Out1/1

== system TIM/Baler/AutoCfg_2 Subsystem/CalcTargetSpeed ==
  SwathVolFlowaRate : Inport
  MATLAB Function : MATLAB Function  TreatAsAtomicUnit=on
  Out2 : Outport
  wires:
  MATLAB Function/1(TargetSpeed) -> Out2/1
  SwathVolFlowaRate/1 -> MATLAB Function/1(u)

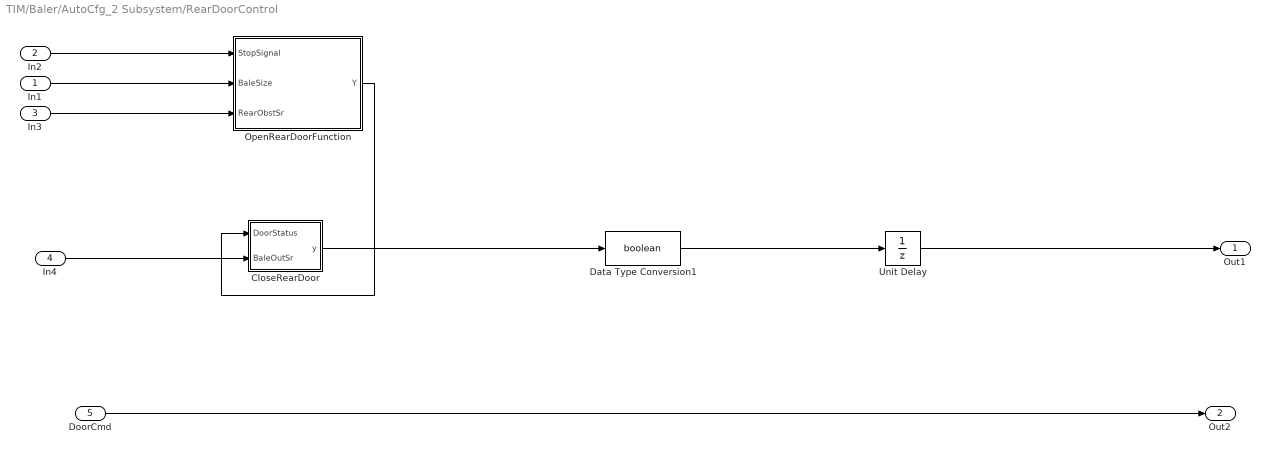
== system TIM/Baler/AutoCfg_2 Subsystem/RearDoorControl ==
  In1 : Inport
  In2 : Inport  Port=2
  In3 : Inport  Port=3
  In4 : Inport  Port=4
  DoorCmd : Inport  Port=5
  CloseRearDoor : MATLAB Function  TreatAsAtomicUnit=on
  Data Type Conversion1 : DataTypeConversion  OutDataTypeStr=boolean
  OpenRearDoorFunction : MATLAB Function  TreatAsAtomicUnit=on
  Unit Delay : UnitDelay  SampleTime=-1
  Out1 : Outport
  Out2 : Outport  Port=2
  wires:
  Unit Delay/1 -> Out1/1
  DoorCmd/1 -> Out2/1
  In4/1 -> CloseRearDoor/2(BaleOutSr)
  In2/1 -> OpenRearDoorFunction/1(StopSignal)
  In1/1 -> OpenRearDoorFunction/2(BaleSize)
  Data Type Conversion1/1 -> Unit Delay/1
  OpenRearDoorFunction/1(Y) -> CloseRearDoor/1(DoorStatus)
  In3/1 -> OpenRearDoorFunction/3(RearObstSr)
  CloseRearDoor/1(y) -> Data Type Conversion1/1

== system TIM/Baler/SemiAutoCfg Subsystem/CalcTargetSpeed ==
  SwathVolFlowaRate : Inport
  MATLAB Function : MATLAB Function  TreatAsAtomicUnit=on
  Out2 : Outport
  wires:
  SwathVolFlowaRate/1 -> MATLAB Function/1(u)
  MATLAB Function/1(TargetSpeed) -> Out2/1

== system TIM/Baler/SemiAutoCfg Subsystem/RearDoorControl ==
  In1 : Inport
  In2 : Inport  Port=2
  In3 : Inport  Port=3
  In4 : Inport  Port=4
  DoorCmd : Inport  Port=5
  CloseRearDoor : MATLAB Function  TreatAsAtomicUnit=on
  Data Type Conversion1 : DataTypeConversion  OutDataTypeStr=boolean
  OpenRearDoorFunction : MATLAB Function  TreatAsAtomicUnit=on
  Unit Delay : UnitDelay  SampleTime=-1
  Out1 : Outport
  Out2 : Outport  Port=2
  wires:
  CloseRearDoor/1(y) -> Data Type Conversion1/1
  In3/1 -> OpenRearDoorFunction/3(RearObstSr)
  OpenRearDoorFunction/1(Y) -> CloseRearDoor/1(DoorStatus)
  Data Type Conversion1/1 -> Unit Delay/1
  In1/1 -> OpenRearDoorFunction/2(BaleSize)
  In2/1 -> OpenRearDoorFunction/1(StopSignal)
  In4/1 -> CloseRearDoor/2(BaleOutSr)
  DoorCmd/1 -> Out2/1
  Unit Delay/1 -> Out1/1

== system TIM/SwathScanner/Auto_1_Cfg Subsystem/CalcVolFlowRate 1 ==
  CurrentSpeed : Inport
  SwathArea : Inport  Port=2
  MATLAB Function : MATLAB Function  TreatAsAtomicUnit=on
  Out1 : Outport
  wires:
  MATLAB Function/1(y) -> Out1/1
  SwathArea/1 -> MATLAB Function/2(area)
  CurrentSpeed/1 -> MATLAB Function/1(speed)

== system TIM/SwathScanner/Auto_2_Cfg&&SemiAuto Subsystem/CalcVolFlowRate 1 ==
  CurrentSpeed : Inport
  SwathArea : Inport  Port=2
  MATLAB Function : MATLAB Function  TreatAsAtomicUnit=on
  Out1 : Outport
  wires:
  CurrentSpeed/1 -> MATLAB Function/1(speed)
  SwathArea/1 -> MATLAB Function/2(area)
  MATLAB Function/1(y) -> Out1/1

== system TIM/SwathScanner/Manual_Cfg Subsystem/CalcVolFlowRate 1 ==
  CurrentSpeed : Inport
  SwathArea : Inport  Port=2
  MATLAB Function : MATLAB Function  TreatAsAtomicUnit=on
  Out1 : Outport
  wires:
  MATLAB Function/1(y) -> Out1/1
  SwathArea/1 -> MATLAB Function/2(area)
  CurrentSpeed/1 -> MATLAB Function/1(speed)

== system TIM/Tractor/Auto_Cfg SubSystem/SpeedController ==
  In1 : Inport
  In2 : Inport  Port=2
  In3 : Inport  Port=3
  In4 : Inport  Port=4
  Constant : Constant  Value=0
  Constant1 : Constant
  Switch2 : Switch  Criteria=u2 ~= 0  Threshold=2
  setSpeed : MATLAB Function  TreatAsAtomicUnit=on
  Out1 : Outport
  Out2 : Outport  Port=2
  wires:
  In2/1 -> setSpeed/2(Tspeed)
  Constant/1 -> Switch2/1
  Constant1/1 -> Switch2/3
  In1/1 -> setSpeed/1(Cspeed)
  setSpeed/1(y) -> Out1/1, Switch2/2
  In4/1 -> setSpeed/3(BaleSize)
  Switch2/1 -> Out2/1
  In3/1 -> setSpeed/4(FrontObstSr)

== system TIM/Tractor/Auto_Cfg SubSystem/ValveController ==
  In1 : Inport
  Constant : Constant
  Constant1 : Constant  Value=0
  Data Type Conversion : DataTypeConversion  OutDataTypeStr=boolean
  Switch : Switch  Criteria=u2 ~= 0
  Out1 : Outport
  wires:
  In1/1 -> Switch/2
  Switch/1 -> Data Type Conversion/1
  Constant1/1 -> Switch/3
  Constant/1 -> Switch/1
  Data Type Conversion/1 -> Out1/1

== system TIM/Tractor/ManualCfg SubSystem/SpeedController ==
  In1 : Inport
  In2 : Inport  Port=2
  Stop : Inport  Port=3
  Constant : Constant  Value=0
  Constant1 : Constant
  Switch2 : Switch  Criteria=u2 ~= 0  Threshold=2
  setSpeed : MATLAB Function  TreatAsAtomicUnit=on
  Out1 : Outport
  Out2 : Outport  Port=2
  wires:
  In2/1 -> setSpeed/2(SpBedalAngl)
  Constant/1 -> Switch2/1
  Constant1/1 -> Switch2/3
  In1/1 -> setSpeed/1(Cspeed)
  setSpeed/1(y) -> Out1/1, Switch2/2
  Switch2/1 -> Out2/1
  Stop/1 -> setSpeed/3(StopReq)

== system TIM/Tractor/ManualCfg SubSystem/ValveController ==
  In1 : Inport
  Constant : Constant
  Constant1 : Constant  Value=0
  Data Type Conversion : DataTypeConversion  OutDataTypeStr=boolean
  Switch : Switch  Criteria=u2 ~= 0
  Out1 : Outport
  wires:
  In1/1 -> Switch/2
  Switch/1 -> Data Type Conversion/1
  Constant1/1 -> Switch/3
  Constant/1 -> Switch/1
  Data Type Conversion/1 -> Out1/1

== system TIM/Tractor/SemiAuto_Cfg SubSystem/SpeedController ==
  In1 : Inport
  In2 : Inport  Port=2
  In3 : Inport  Port=3
  In4 : Inport  Port=4
  Constant : Constant  Value=0
  Constant1 : Constant
  Switch2 : Switch  Criteria=u2 ~= 0  Threshold=2
  setSpeed : MATLAB Function  TreatAsAtomicUnit=on
  Out1 : Outport
  Out2 : Outport  Port=2
  wires:
  In3/1 -> setSpeed/4(FrontObstSr)
  Switch2/1 -> Out2/1
  In4/1 -> setSpeed/3(BaleSize)
  setSpeed/1(y) -> Switch2/2, Out1/1
  In1/1 -> setSpeed/1(Cspeed)
  Constant1/1 -> Switch2/3
  Constant/1 -> Switch2/1
  In2/1 -> setSpeed/2(Tspeed)

== system TIM/Tractor/SemiAuto_Cfg SubSystem/ValveController ==
  In1 : Inport
  Constant : Constant
  Constant1 : Constant  Value=0
  Data Type Conversion : DataTypeConversion  OutDataTypeStr=boolean
  Switch : Switch  Criteria=u2 ~= 0
  Out1 : Outport
  wires:
  Data Type Conversion/1 -> Out1/1
  Constant/1 -> Switch/1
  Constant1/1 -> Switch/3
  Switch/1 -> Data Type Conversion/1
  In1/1 -> Switch/2

== matlab function TIM/Tractor/Auto_Cfg SubSystem/SpeedController/setSpeed ==
  data: Cspeed input; y output; Tspeed input; BaleSize input; FrontObstSr input
function y = fcn(Cspeed, Tspeed,BaleSize, FrontObstSr)

if(BaleSize==2 || FrontObstSr==1)
    y = (Cspeed-(Cspeed-Tspeed))*0;


elseif(BaleSize==1)
y = ((Cspeed-(Cspeed-Tspeed))*0.50);
else
   y = (Cspeed-(Cspeed-Tspeed)); 
end

== matlab function TIM/Baler/AutoCfg_1 SubSystem/CalcTargetSpeed/MATLAB Function ==
  data: u input; TargetSpeed output
function TargetSpeed = fcn(u)

  
TargetSpeed = -.10*u+20;
end

== matlab function TIM/SwathScanner/Manual_Cfg Subsystem/CalcVolFlowRate 1/MATLAB Function ==
  data: speed input; y output; area input
function y = fcn(speed, area)

y = speed*area;

== matlab function TIM/Baler/AutoCfg_1 SubSystem/RearDoorControl/OpenRearDoorFunction ==
  data: StopSignal input; Y output; BaleSize input; RearObstSr input

function Y = fcn(StopSignal,BaleSize,RearObstSr)

if (StopSignal==1 && BaleSize==2 && RearObstSr==0)
    Y =1;
else
    
    Y=0;
    
end

== matlab function TIM/Baler/AutoCfg_1 SubSystem/RearDoorControl/CloseRearDoor ==
  data: DoorStatus input; y output; BaleOutSr input
function y = fcn(DoorStatus, BaleOutSr)
if (DoorStatus==1 &&BaleOutSr==1)
y = 0;
else
 y=DoorStatus;
    
end

== matlab function TIM/Baler/AutoCfg_1 SubSystem/CalcTargetAngel ==
  data: SWL input; TargetAngle output
function TargetAngle = fcn(SWL)

  
TargetAngle = 3*SWL;
end

== stateflow chart TIM/Baler/BalerMode1 ==
  state SensorsLogic [parallel]
    settings: executionOrder=1
    state BothSrsWork
      entry: BalerMode=3;
      SysReconfigReq=0;
    state FirstSrFail
      entry:  BalerMode=3.2;
      SysReconfigReq=0;
    state BotheFail
      entry:  BalerMode=1;
      SysReconfigReq=1;
    state SecondSrFail [commented out]
      entry:  BalerMode=2;
      SysReconfigReq=1.2;
    BothSrsWork -> FirstSrFail : [RObstSr_isBroken(RSr1) ]
    (default) -> BothSrsWork
    FirstSrFail -> BothSrsWork [order 2] : [~(RObstSr_isBroken(RSr1))]
    BothSrsWork -> SecondSrFail [commented out] : [RObstSr_isBroken(RSr2)]
    SecondSrFail -> BothSrsWork [commented out] : [~RObstSr_isBroken(RSr2)]
    BotheFail -> BothSrsWork [order 1] : [~(RObstSr_isBroken(RSr1))&&~(RObstSr_isBroken(RSr2))]
    BotheFail -> FirstSrFail [order 2] : [~(RObstSr_isBroken(RSr2))]
    FirstSrFail -> BotheFail [order 1] : [(RObstSr_isBroken(RSr2))]
    SecondSrFail -> BotheFail [commented out] : [RObstSr_isBroken(RSr1)]
    BotheFail -> SecondSrFail [commented out] : [~RObstSr_isBroken(RSr1)]
  state BalerLogic [parallel]
    settings: executionOrder=2
    state Auto
      entry: SysModeOut=3 ;
      ِ
      state Auto3
        entry:BalerCfgMode=3.2;
        AutoCfg_2=true;
        exit:AutoCfg_2=false;
      state Auto1
        entry:BalerCfgMode=3.1;
        AutoCfg_1=true;
        exit:AutoCfg_1=false;
        ِ
      Auto1 -> Auto3 : [ BalerMode==3.2]
      (default) -> Auto1
    state SemiAuto
      entry: SysModeOut=2;
      BalerCfgMode=2;
      SemiAutoCfg=true;
      exit:SemiAutoCfg=false;
    state Manual
      entry: SysModeOut=1;
      BalerCfgMode=1;
    Manual -> Auto [order 2] : [ModeInput==3]
    Manual -> SemiAuto [order 1] : [ModeInput==2&&(BalerMode~=1)]
    (default) -> Manual
    SemiAuto -> Auto [order 1] : [ModeInput==3]
    SemiAuto -> Manual [order 2] : [ModeInput==1]
    Auto -> SemiAuto [order 3] : [ModeInput==2]
    Auto -> Manual [order 1] : [ModeInput==1]
    Auto -> SemiAuto [order 2] : [( ModeInput==2)]
  data: obst function_input; status function_output; ModeInput input; SysModeOut output; RSr1 input; RSr2 input; BalerCfgMode output; SysReconfigReq output; AutoCfg_1 output; AutoCfg_2 output; SemiAutoCfg output; BalerMode local
  function status=RObstSr_isBroken(obst):
    | function status=RObstSr_isBroken(obst)
    |  
    | if ((obst==1)||(obst==0))
    | 
    | status=false;
    | else
    |     status=true;
    | end

== stateflow chart TIM/Tractor/TractorMode ==
  state Manual
    entry: SysModeOut=1;
    ManualCfg=true;
    exit:ManualCfg=false;
  state SemiAuto
    entry: SysModeOut=2;
    SemiAutoCfg=true;
    exit:SemiAutoCfg=false;
  state Auto
    entry: SysModeOut=3;
    AutoCfg=true;
    exit:AutoCfg=false;
  Manual -> Auto [order 2] : [(ModeInput==3)&&(SysReconfigReq~=1)]
  Auto -> SemiAuto [order 2] : [(ModeInput==2) || (FrontObsSr_isBroken(Fobst))]{ AutoCfg=false}
  (default) -> Manual
  Manual -> SemiAuto [order 1] : [ModeInput==2&&((SysReconfigReq~=1)&&(SysReconfigReq~=1.2))]
  SemiAuto -> Manual [order 2] : [(ModeInput==1)||(SysReconfigReq==1.2)]
  SemiAuto -> Auto [order 1] : [(ModeInput==3)&&(~FrontObsSr_isBroken(Fobst))]
  Auto -> Manual [order 1] : [(ModeInput==1)||(SysReconfigReq==1)]
  data: FobstValue function_input; status function_output; ModeInput input; SysModeOut output; Fobst input; AutoCfg output boolean; SemiAutoCfg output boolean; ManualCfg output boolean; SysReconfigReq input
  function status = FrontObsSr_isBroken(FobstValue):
    | function status=FrontObsSr_isBroken(FobstValue)
    | 
    | if ((FobstValue==1)||(FobstValue==0))
    | 
    | status=false;
    | else
    |     status=true;
    | end

== stateflow chart TIM/Baler/BalerMode ==
  state Auto
    entry: SysModeOut=3 ;
    ِ
    state Auto3
      entry:BalerCfgMode=3.2;
      AutoCfg_2=true;
      exit:AutoCfg_2=false;
    state Auto1
      entry:BalerCfgMode=3.1;
      AutoCfg_1=true;
      exit:AutoCfg_1=false;
      ِ
    Auto1 -> Auto3 : [RObstSr_isBroken(RSr1)]
    (default) -> Auto1
  state Manual
    entry: SysModeOut=1;
    BalerCfgMode=1;
  state SemiAuto
    entry: SysModeOut=2;
    BalerCfgMode=2;
    SemiAutoCfg=true;
    exit:SemiAutoCfg=false;
  state interReconfigState
    entry:
    BalerCfgMode=0;
    SysReconfigReq=1;
    exit: SysReconfigReq=-1;
    note: coz baler cant independently reconfig intraRecfg
  Manual -> Auto [order 2] : [ModeInput==3]
  Manual -> SemiAuto [order 1] : [ModeInput==2]
  (default) -> Manual
  SemiAuto -> Auto [order 1] : [ModeInput==3]
  SemiAuto -> Manual [order 2] : [ModeInput==1]
  Auto -> Manual [order 1] : [ModeInput==1]
  interReconfigState -> Manual [order 2] : [( ModeInput==1)]
  Auto -> SemiAuto [order 3] : [ModeInput==2]
  interReconfigState -> SemiAuto [order 1] : [( ModeInput==2)]
  Auto -> interReconfigState [order 2] : [((RObstSr_isBroken(RSr1))&&(RObstSr_isBroken(RSr2)))]
  data: obst function_input; status function_output; ModeInput input; SysModeOut output; RSr1 input; RSr2 input; BalerCfgMode output; SysReconfigReq output; AutoCfg_1 output; AutoCfg_2 output; SemiAutoCfg output
  function status=RObstSr_isBroken(obst):
    | function status=RObstSr_isBroken(obst)
    |  
    | if ((obst==1)||(obst==0))
    | 
    | status=false;
    | else
    |     status=true;
    | end

== stateflow chart TIM/SwathScanner/Chart ==
  state AutoCfg
    state Auto1
      entry: SysModeOut=3.1;
      AutoCfg1=true;
      exit: AutoCfg1=false;
    state Auto2
      entry: SysModeOut=3.2;
      AutoCfg2=true;
      exit:AutoCfg2=false;
    (default) -> (junction 63) [commented out]
    (junction 63) -> Auto2 [commented out] : [isBroken(SpSr1)==true]
    (junction 63) -> Auto1 [commented out] : [[isBroken(SpSr1)==false]]
    Auto1 -> Auto2 : [isBroken(SpSr1)==true]
    (default) -> Auto1
  state SemiAuto
    entry: SysModeOut=2;
    AutoCfg2=true;
    exit:AutoCfg2=false;
  state Manual
    entry: SysModeOut=1;
    ManualCfg=true;
    exit:ManualCfg=false;
  Manual -> AutoCfg [order 2] : [ModeInput==3]
  AutoCfg -> SemiAuto [order 1] : [ModeInput==2]
  Manual -> SemiAuto [order 1] : [ModeInput==2]
  (default) -> Manual
  SemiAuto -> AutoCfg [order 1] : [ModeInput==3]
  SemiAuto -> Manual [order 2] : [ModeInput==1]
  AutoCfg -> Manual [order 2] : [ModeInput==1]
  data: Speed function_input; status function_output; ModeInput input; SysModeOut output; AutoCfg1 output boolean; AutoCfg2 output boolean; SpSr1 input; ManualCfg output boolean
  function status=isBroken(Speed):
    | function status=isBroken(Speed)
    | 
    | if ((Speed>20)||(Speed<0))
    | 
    | status=true;
    | else
    |     status=false;
    | end

== matlab function TIM/SwathScanner/Auto_1_Cfg Subsystem/CalcVolFlowRate 1/MATLAB Function ==
  data: speed input; y output; area input
function y = fcn(speed, area)

y = speed*area;

== matlab function TIM/SwathScanner/Auto_2_Cfg&&SemiAuto Subsystem/CalcVolFlowRate 1/MATLAB Function ==
  data: speed input; y output; area input
function y = fcn(speed, area)

y = speed*area;

== matlab function TIM/Tractor/SemiAuto_Cfg SubSystem/SpeedController/setSpeed ==
  data: Cspeed input; y output; Tspeed input; BaleSize input; FrontObstSr input
function y = fcn(Cspeed, Tspeed,BaleSize, FrontObstSr)

if(BaleSize==2 || FrontObstSr==1)
    y = (Cspeed-(Cspeed-Tspeed))*0;


elseif(BaleSize==1)
y = ((Cspeed-(Cspeed-Tspeed))*0.50);
else
   y = (Cspeed-(Cspeed-Tspeed)); 
end

== matlab function TIM/Tractor/ManualCfg SubSystem/SpeedController/setSpeed ==
  data: Cspeed input; y output; SpBedalAngl input; StopReq input
function y = fcn(Cspeed, SpBedalAngl, StopReq)

if(StopReq==1)
    y = 0;
else
   y = (Cspeed-(Cspeed-(4*SpBedalAngl))); 
end
